simulink model "Problem_1"  (R2020a)
settings: Solver=VariableStepAuto  StartTime=0.0  StopTime=10.0  RelTol=1e-3
settings Model: Creator=Admin  LastModifiedBy=Admin

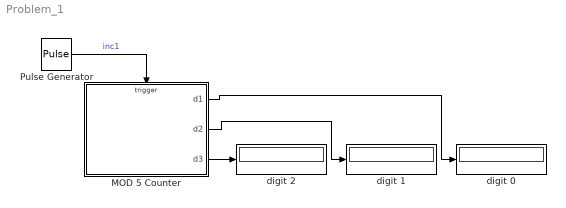
== system Problem_1 ==
  MOD 5 Counter : Stateflow chart  TreatAsAtomicUnit=on
  Pulse Generator : DiscretePulseGenerator  PulseType=Time based  Period=0.01  PulseWidth=5  PhaseDelay=0.1
  digit 0 : Display
  digit 1 : Display
  digit 2 : Display
  wires:
  MOD 5 Counter/1(d1) -> digit 0/1
  MOD 5 Counter/3(d3) -> digit 2/1
  Pulse Generator/1 -> MOD 5 Counter/Trigger  "inc1"
  MOD 5 Counter/2(d2) -> digit 1/1

== stateflow chart Problem_1/MOD 5 Counter ==
  settings: executeAtInitialization=1
  state digit1 [parallel]
    settings: executionOrder=1
    state one
      en:
      d1=1;
    state zero
      en:
      d1=0;
    state two
      en:
      d1=2;
    state four
      en:
      d1=4;
    state three
      en:
      d1=3;
    (default) -> digit1.zero
    digit1.zero -> digit1.one : inc1
    digit1.one -> digit1.two : inc1
    digit1.two -> digit1.three : inc1
    digit1.four -> digit1.zero : inc1/{inc2;}
    digit1.three -> digit1.four : inc1
  state digit2 [parallel]
    settings: executionOrder=2
    state one
      en:
      d2=1;
    state two
      en:
      d2=2;
    state zero
      en:
      d2=0;
    state three
      en:
      d2=3;
    state four
      en:
      d2=4;
    digit2.one -> digit2.two : inc2
    (default) -> digit2.zero
    digit2.zero -> digit2.one : inc2
    digit2.two -> digit2.three : inc2
    digit2.four -> digit2.zero : inc2/{inc3;}
    digit2.three -> digit2.four : inc2
  state digit3 [parallel]
    settings: executionOrder=3
    state one
      en:
      d3=1;
    state two
      en:
      d3=2;
    state zero
      en:
      d3 = 0;
    state four
      en:
      d3=4;
    state three
      en:
      d3=3;
    (default) -> digit3.zero
    digit3.one -> digit3.two : inc3
    digit3.zero -> digit3.one : inc3
    digit3.four -> digit3.zero : inc3
    digit3.two -> digit3.three : inc3
    digit3.three -> digit3.four : inc3
  data: d1 output size=1; d2 output size=1; d3 output size=1
  events: inc3 local FUNCTION_CALL_EVENT; inc2 local RISING_EDGE_EVENT; inc1 input RISING_EDGE_EVENT
